simulink model "Accelerometer"  (R2018a)
settings: Solver=ode15s  StartTime=0.0  StopTime=0.25  RelTol=1e-3  EnableMultiTasking=on
values from neighbouring files (symbols this model uses):
  A = 24*10^(-6)    (= 2.4e-05)    [AccData.m]
  C_0 = 10.6e-12    (= 1.06e-11)    [AccData.m]
  C_3 = 1e-9    (= 1e-09)    [AccData.m]
  C_4 = 22e-12    (= 2.2e-11)    [AccData.m]
  d0 = 10^(-5)    (= 1e-05)    [AccData.m]
  den_1 = R_7*R_8*R_9*C_5*C_6    (= 0.000729)    [AccData.m]
  den_2 = C_6*(R_7+R_8)-C_5*R_7*R_10/R_9    (= 0.0003888)    [AccData.m]
  eps0 = 8.854*10^(-12)    (= 8.854e-12)    [AccData.m]
  k = 83.3    [AccData.m]
  m = 8.2*10^(-6)    (= 8.2e-06)    [AccData.m]
  num_1 = 1+R_10/R_9    (= 1.56)    [AccData.m]
  R_1 = 250e6    (= 250000000)    [AccData.m]
  R_2 = 820e3    (= 820000)    [AccData.m]
settings Model: Creator=Valentin  LastModifiedBy=Mihaela
settings DataIOCC: LimitDataPoints=on  SaveFormat=Array  SignalLoggingSaveFormat=ModelDataLogs
settings OptimizationCC: ExpressionDepthLimit=2147483647  InitFltsAndDblsToZero=on  LifeSpan=inf
settings DebuggingCC: UnderspecifiedInitializationDetection=Classic  MergeDetectMultiDrivingBlocksExec=none  SolverPrmCheckMsg=warning  FcnCallInpInsideContextMsg=warning  StateNameClashWarn=warning  LibraryContextMissingDiagnostic=warning  SFUnexpectedBacktrackingDiag=warning  SFNoUnconditionalDefaultTransitionDiag=warning  SFExecutionAtInitializationDiag=none
settings HardwareCC: ProdBitPerPointer=32  ProdBitPerSizeT=32  ProdBitPerPtrDiffT=32  ProdLargestAtomicFloat=None  ProdIntDivRoundTo=Undefined  ProdEndianess=Unspecified  ProdWordSize=32  ProdHWDeviceType=32-bit Generic
settings ModelReferenceCC: PropagateSignalLabelsOutOfModel=off
settings CodeAppCC: StateflowObjectComments=on
settings GRTTargetCC: TargetLangStandard=C89/C90 (ANSI)  GeneratePreprocessorConditionals=Disable all  CombineOutputUpdateFcns=off  GRTInterface=on
settings ConfigComp: CovMetricSettings=dw  CovHtmlReporting=on  CovSaveCumulativeToWorkspaceVar=on  CovSaveSingleToWorkspaceVar=on  CovExternalEMLEnable=off

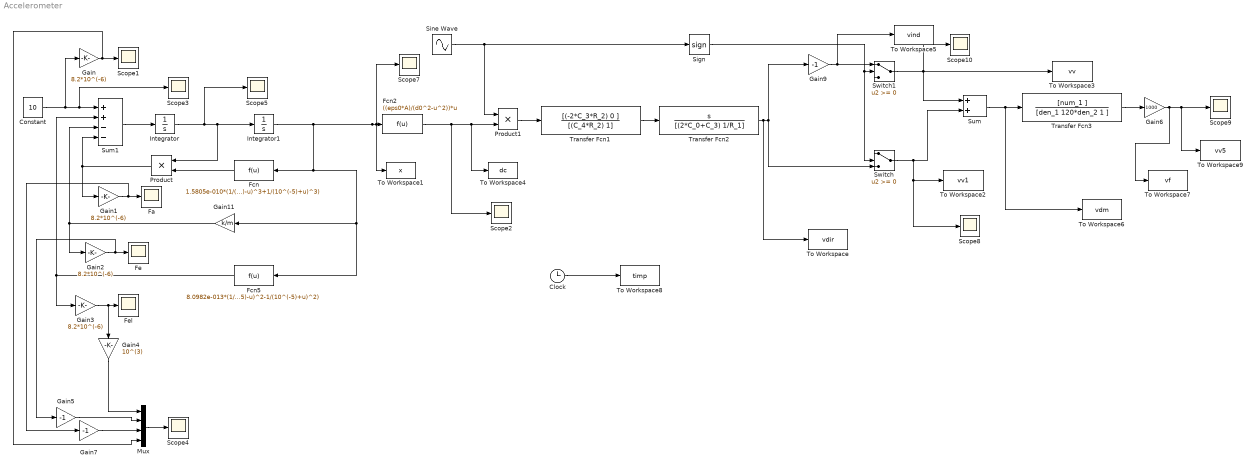
== system Accelerometer ==
  Clock : Clock
  Constant : Constant  Value=10
  Fa : Scope
  Fcn : Fcn  Expr=1.5805e-010*(1/(10^(-5)-u)^3+1/(10^(-5)+u)^3)
  Fcn2 : Fcn  Expr=((eps0*A)/(d0^2-u^2))*u
  Fcn5 : Fcn  Expr=8.0982e-013*(1/(10^(-5)-u)^2-1/(10^(-5)+u)^2)
  Fe : Scope
  Fel : Scope
  Gain{,1..3} (4 alike) : Gain  Gain=8.2*10^(-6)
  Gain11 : Gain  Gain=k/m
  Gain4 : Gain  Gain=10^(3)
  Gain5 : Gain  Gain=-1
  Gain6 : Gain  Gain=1000
  Gain7 : Gain  Gain=-1
  Gain9 : Gain  Gain=-1
  Integrator : Integrator
  Integrator1 : Integrator
  Mux : Mux
  Product : Product  RndMeth=Zero
  Product1 : Product  RndMeth=Zero
  Scope{1..5,7..10} (9 alike) : Scope
  Sign : Signum
  Sine Wave : Sin  Amplitude=0.5  Frequency=10000  SampleTime=0
  Sum : Sum
  Sum1 : Sum  Inputs=++--
  Switch : Switch
  Switch1 : Switch
  To Workspace : ToWorkspace  VariableName=vdir  SaveFormat=Timeseries  SampleTime=-1
  To Workspace1 : ToWorkspace  VariableName=x  SaveFormat=Timeseries  SampleTime=-1
  To Workspace2 : ToWorkspace  VariableName=vv1  SampleTime=-1
  To Workspace3 : ToWorkspace  VariableName=vv  SampleTime=-1
  To Workspace4 : ToWorkspace  VariableName=dc  SaveFormat=Timeseries  SampleTime=-1
  To Workspace5 : ToWorkspace  VariableName=vind  SaveFormat=Timeseries  SampleTime=-1
  To Workspace6 : ToWorkspace  VariableName=vdm  SaveFormat=Timeseries  SampleTime=-1
  To Workspace7 : ToWorkspace  VariableName=vf  SaveFormat=Timeseries  SampleTime=-1
  To Workspace8 : ToWorkspace  VariableName=timp  SampleTime=-1
  To Workspace9 : ToWorkspace  VariableName=vv5  SampleTime=-1
  Transfer Fcn1 : TransferFcn  Numerator=[(-2*C_3*R_2) 0 ]  Denominator=[(C_4*R_2) 1]
  Transfer Fcn2 : TransferFcn  Numerator=[1 0]  Denominator=[(2*C_0+C_3) 1/R_1]
  Transfer Fcn3 : TransferFcn  Numerator=[num_1 ]  Denominator=[den_1 120*den_2 1 ]
  wires:
  Constant/1 -> Gain/1, Sum1/1, Scope3/1
  Sum1/1 -> Integrator/1
  Integrator/1 -> Integrator1/1, Product/1, Scope5/1
  Integrator1/1 -> Fcn5/1, Gain11/1, Fcn/1, Scope7/1, To Workspace1/1, Fcn2/1
  Fcn/1 -> Product/2
  Product/1 -> Sum1/4, Gain1/1
  Gain/1 -> Scope1/1, Mux/4
  Gain1/1 -> Fa/1, Gain7/1
  Gain2/1 -> Fe/1, Gain5/1
  Gain3/1 -> Fel/1, Gain4/1
  Mux/1 -> Scope4/1
  Gain4/1 -> Mux/1
  Gain5/1 -> Mux/2
  Gain7/1 -> Mux/3
  Fcn2/1 -> To Workspace4/1, Product1/2, Scope2/1
  Gain11/1 -> Sum1/3, Gain2/1
  Fcn5/1 -> Sum1/2, Gain3/1
  Sine Wave/1 -> Product1/1, Sign/1
  Product1/1 -> Transfer Fcn1/1
  Gain9/1 -> To Workspace5/1, Switch1/1
  Switch/1 -> Sum/2, Scope8/1, To Workspace2/1
  Sum/1 -> To Workspace6/1, Transfer Fcn3/1
  Sign/1 -> Switch/2, Switch1/2
  Switch1/1 -> Sum/1, To Workspace3/1, Scope10/1
  Clock/1 -> To Workspace8/1
  Transfer Fcn1/1 -> Transfer Fcn2/1
  Transfer Fcn2/1 -> To Workspace/1, Gain9/1, Switch/3
  Transfer Fcn3/1 -> Gain6/1
  Gain6/1 -> To Workspace7/1, Scope9/1, To Workspace9/1
